simulink model "MLIB_RndSat_BAM"  (Simulink 8.3)
settings: Solver=ode45  StartTime=0.0  StopTime=10.0  RelTol=1e-3
settings Model: Creator=B37097  LastModifiedBy=B37097
settings DataIOCC: SignalLoggingSaveFormat=Dataset
settings DebuggingCC: UnderspecifiedInitializationDetection=Simplified  StateNameClashWarn=none
settings GRTTargetCC: CombineOutputUpdateFcns=on  GRTInterface=off

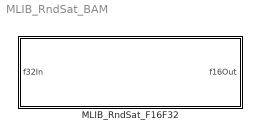
== system MLIB_RndSat_BAM ==
  MLIB_RndSat_F16F32 : Subsystem  mask(MLIB_RndSat_F16F32){}
      mask help: Bit accurate model for conversion of input value. Input parameter is considered as 32-bit integer and output value is considered as 16-bit integer value.
      mask init:
      | pos = get_param(gcb, 'Position');width = pos(3) - pos(1); height = pos(4) - pos(2);tX=width/2;tY=height*0.9;
      mask Display: color('black');port_label('input',1,'f32In');port_label('output',1,'f16Out');color('black');disp('MLIB_RndSat_F16F32');color('blue');text(tX,tY, 'BAM', 'horizontalAlignment', 'center');

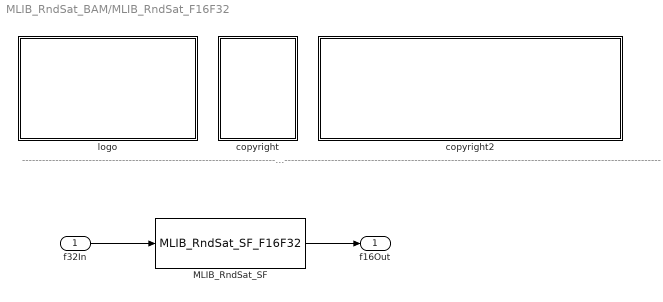
== system MLIB_RndSat_BAM/MLIB_RndSat_F16F32 ==
  note: ---------------------------------------------------------------------------------------------------------------------------------------------------------------------------------------------------
  f32In : Inport
  MLIB_RndSat_SF : S-Function  FunctionName=MLIB_RndSat_SF_F16F32  EnableBusSupport=off
  copyright : Subsystem
      mask Display: text(10,90,'FILE:');text(10,75,'DESRIPTION:');text(10,60,'COPYRIGHT:');text(10,45,'VERSION:');text(10,30,'DATE:')
  copyright2 : Subsystem
      mask Display: text(10,90,'MLIB_RndSat_BAM_F16F32.mdl');text(10,75,'Rounding of the input value to the nearest saturated value in output format.');text(10,60,'Freescale');text(10,45,'1.0');text(10,30,'05-May-2016');
  logo : Subsystem
      mask Display: image(imread('logo.jpg'))
  f16Out : Outport
  wires:
  f32In/1 -> MLIB_RndSat_SF/1
  MLIB_RndSat_SF/1 -> f16Out/1

== system MLIB_RndSat_BAM/MLIB_RndSat_F16F32/copyright ==

== system MLIB_RndSat_BAM/MLIB_RndSat_F16F32/copyright2 ==

== system MLIB_RndSat_BAM/MLIB_RndSat_F16F32/logo ==
